simulink model "gainconstantsubsystem"  (Simulink 6.6)
settings: Solver=FixedStepDiscrete  StartTime=0.0  StopTime=10.0  FixedStep=1  RelTol=1e-3
settings Model: Creator=ksmyth  LastModifiedBy=ksmyth
settings DebuggingCC: SignalResolutionControl=TryResolveAllWithWarning  MultiTaskDSMMsg=warning  MultiTaskCondExecSysMsg=none
settings RTWCC: IncludeERTFirstTime=on

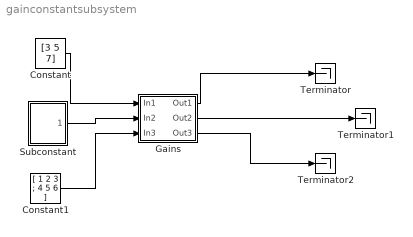
== system gainconstantsubsystem ==
  Constant : Constant  Value=[3 5 7]  VectorParams1D=off
  Constant1 : Constant  Value=[ 1 2 3 ; 4 5 6 ]
  Gains : Subsystem
  Subconstant : Subsystem
  Terminator : Terminator
  Terminator1 : Terminator
  Terminator2 : Terminator
  wires:
  Constant/1 -> Gains/1(In1)
  Gains/1(Out1) -> Terminator/1
  Subconstant/1(Out1) -> Gains/2(In2)
  Gains/2(Out2) -> Terminator1/1
  Gains/3(Out3) -> Terminator2/1
  Constant1/1 -> Gains/3(In3)

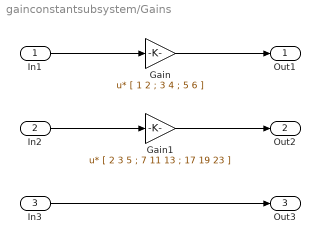
== system gainconstantsubsystem/Gains ==
  In1 : Inport
  In2 : Inport  Port=2
  In3 : Inport  Port=3
  Gain : Gain  Gain=[ 1 2 ; 3 4 ; 5 6 ]  Multiplication=Matrix(u*K)
  Gain1 : Gain  Gain=[ 2 3 5 ; 7 11 13 ; 17 19 23 ]  Multiplication=Matrix(u*K)
  Out1 : Outport
  Out2 : Outport  Port=2
  Out3 : Outport  Port=3
  wires:
  In1/1 -> Gain/1
  Gain/1 -> Out1/1
  In2/1 -> Gain1/1
  Gain1/1 -> Out2/1
  In3/1 -> Out3/1

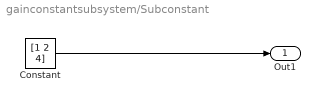
== system gainconstantsubsystem/Subconstant ==
  Constant : Constant  Value=[1 2 4]
  Out1 : Outport
  wires:
  Constant/1 -> Out1/1
